simulink model "ECG_test"  (R2020a)
settings: Solver=FixedStepAuto  StartTime=0.0  StopTime=120  FixedStep=1e-3  RelTol=1e-3  EnableMultiTasking=on
undefined symbols (not defined in the file or in its folder): A3, A4, D0, D1, D10, D11, D12, D13, D2, D3, D5, D6, D8, D9, Modes, PTA0, PTA1, PTA2, PTB11, PTB9, PTC11, PTC16, PTC17, PTC2, PTC4, PTD0, PTD1, PTD2, PTD3
libraries: frdmk64flib x15, simulink x1
settings Model: SimulationMode=external  ExtModeTrigDuration=5  Creator=aboda  LastModifiedBy=USER
settings OptimizationCC: EnhancedBackFolding=on  PassReuseOutputArgsAs=Individual arguments  ZeroExternalMemoryAtStartup=off  ZeroInternalMemoryAtStartup=off  MaxStackSize=64  OptimizeBlockOrder=speed  DifferentSizesBufferReuse=on  OptimizationCustomize=off  EfficientTunableParamExpr=on
settings DebuggingCC: ParameterTunabilityLossMsg=error
settings HardwareCC: ProdBitPerPointer=32  ProdBitPerSizeT=32  ProdBitPerPtrDiffT=32  ProdLargestAtomicInteger=Long  ProdLargestAtomicFloat=Double  ProdWordSize=32  ProdHWDeviceType=ARM Compatible->ARM Cortex
settings SFSimCC: MATLABDynamicMemAlloc=off
settings RTWCC: SystemTargetFile=ert.tlc  HardwareBoard=NXP FRDM-K64F  TemplateMakefile=ert_default_tmf  Toolchain=GNU Tools for ARM Embedded Processors
settings CodeAppCC: ForceParamTrailComments=on  IgnoreCustomStorageClasses=off  OperatorAnnotations=on  SimulinkDataObjDesc=on  SFDataObjDesc=on  InsertBlockDesc=on
settings ERTTargetCC: ExtMode=on  ExtModeTransport=4  ExtModeMexFile=sendToCommService  ExtModeMexArgs='ECG_test' 0

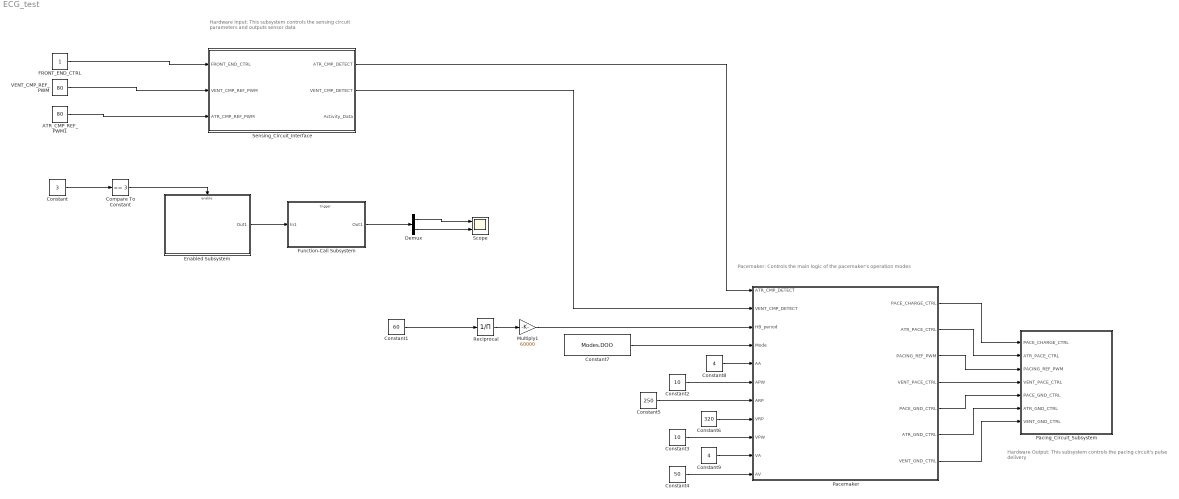
== system ECG_test ==
  note: Hardware Output: This subsystem controls the pacing circuit's pulse delivery
  note: Pacemaker: Controls the main logic of the pacemaker's operation modes
  note: Hardware Input: This subsystem controls the sensing circuit parameters and outputs sensor data
  ATR_CMP_REF_PWM1 : Constant  Value=80  OutDataTypeStr=uint8
  Compare To Constant : simulink/Logic and Bit Operations/Compare To Constant  relop===  const=3  OutDataTypeStr=boolean
  Constant : Constant  Value=3
  Constant1 : Constant  Value=60  OutDataTypeStr=uint8
  Constant2 : Constant  Value=10  OutDataTypeStr=uint8
  Constant3 : Constant  Value=10  OutDataTypeStr=uint8
  Constant4 : Constant  Value=50  OutDataTypeStr=uint16
  Constant5 : Constant  Value=250  OutDataTypeStr=uint16
  Constant6 : Constant  Value=320  OutDataTypeStr=uint16
  Constant7 : Constant  Value=Modes.DOO  OutDataTypeStr=Enum: Modes
  Constant8 : Constant  Value=4  OutDataTypeStr=single
  Constant9 : Constant  Value=4  OutDataTypeStr=single
  Demux : Demux  Outputs=2
  Enabled Subsystem : Subsystem  TreatAsAtomicUnit=on
  FRONT_END_CTRL : Constant  OutDataTypeStr=boolean
  Function-Call Subsystem : Subsystem  TreatAsAtomicUnit=on
  Multiply1 : Gain  Gain=60000  OutDataTypeStr=uint16  RndMeth=Round  SaturateOnIntegerOverflow=on
  Pacemaker : Stateflow chart  TreatAsAtomicUnit=on
      settings: PortSchema="{\"entries\":[{\"content\":{\"sides\":[{\"content\":{\"connectorIds\":[\"In2\",\"In3\",\"In10\",\"In1\",\"In6\",\"In8\",\"In4\",\"In5\",\"In9\",\"In7\",\"In11\"]},\"type\":\"ConnectorPlacement.EquallySpacedRectSide\",\"uuid\":\"be11ab42-f218-4533-b046-48d6c6672980\"},{\"content\":{\"connectorIds\":[\"Out1\",\"Out2\",\"Out3\",\"Out4\",\"Out5\",\"Out6\",\"Out7\"],\"side\":\"RIGHT\"},\"type\":\"ConnectorPlacement.EquallySpacedRectSide\",\"uuid\":\"3184d97a-d95e-4f92-be49-d512e0e8be59\"},{\"content\":{\"connectorIds\":[],\"side\":\"TOP\"},\"type\":\"ConnectorPlacement.EquallySpacedRectSide\",\"uuid\":\"82a667a0-8f6e-4fe8-9d7d-d285af85bcaa\"}]},\"type\":\"ConnectorPlacement.EquallySpacedConnector\",\"uuid\":\"8df3a08e-b350-4a50-854d-64d5d1a667ae\"}],\"packageUris\":[\"http://schema.mathworks.com/mf0/Connector/19700101\"],\"version\":\"1.0\"}"
  Pacing_Circuit_Subsystem : Subsystem
  Reciprocal : Product  Inputs=/  OutDataTypeStr=double  RndMeth=Nearest
  Scope : Scope  NumInputPorts=2
  Sensing_Circuit_Interface : Subsystem
  VENT_CMP_REF_PWM : Constant  Value=80  OutDataTypeStr=uint8
  wires:
  Compare To Constant/1 -> Enabled Subsystem/Enable
  Constant/1 -> Compare To Constant/1
  Enabled Subsystem/1(Out1) -> Function-Call Subsystem/1(In1)
  Function-Call Subsystem/1(Out1) -> Demux/1
  Demux/1 -> Scope/1
  Demux/2 -> Scope/2
  Pacemaker/5(PACE_GND_CTRL) -> Pacing_Circuit_Subsystem/5(PACE_GND_CTRL)
  Pacemaker/1(PACE_CHARGE_CTRL) -> Pacing_Circuit_Subsystem/1(PACE_CHARGE_CTRL)
  Pacemaker/7(VENT_GND_CTRL) -> Pacing_Circuit_Subsystem/7(VENT_GND_CTRL)
  Pacemaker/6(ATR_GND_CTRL) -> Pacing_Circuit_Subsystem/6(ATR_GND_CTRL)
  Pacemaker/4(VENT_PACE_CTRL) -> Pacing_Circuit_Subsystem/4(VENT_PACE_CTRL)
  Pacemaker/2(ATR_PACE_CTRL) -> Pacing_Circuit_Subsystem/2(ATR_PACE_CTRL)
  Pacemaker/3(PACING_REF_PWM) -> Pacing_Circuit_Subsystem/3(PACING_REF_PWM)
  ATR_CMP_REF_PWM1/1 -> Sensing_Circuit_Interface/3(ATR_CMP_REF_PWM)
  VENT_CMP_REF_PWM/1 -> Sensing_Circuit_Interface/2(VENT_CMP_REF_PWM)
  FRONT_END_CTRL/1 -> Sensing_Circuit_Interface/1(FRONT_END_CTRL)
  Sensing_Circuit_Interface/1(ATR_CMP_DETECT) -> Pacemaker/2(ATR_CMP_DETECT)
  Sensing_Circuit_Interface/2(VENT_CMP_DETECT) -> Pacemaker/3(VENT_CMP_DETECT)
  Constant3/1 -> Pacemaker/9(VPW)
  Constant4/1 -> Pacemaker/11(AV)
  Constant5/1 -> Pacemaker/4(ARP)
  Constant6/1 -> Pacemaker/5(VRP)
  Constant2/1 -> Pacemaker/8(APW)
  Constant7/1 -> Pacemaker/1(Mode)
  Constant8/1 -> Pacemaker/6(AA)
  Constant9/1 -> Pacemaker/7(VA)
  Reciprocal/1 -> Multiply1/1
  Constant1/1 -> Reciprocal/1
  Multiply1/1 -> Pacemaker/10(HB_period)

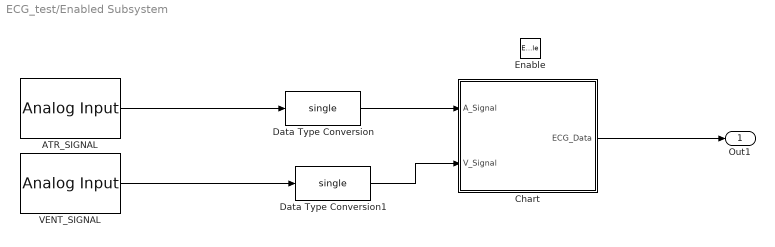
== system ECG_test/Enabled Subsystem ==
  Enable : EnablePort
  ATR_SIGNAL : frdmk64flib/Analog Input  Whichpin=PTB11 (A3)  SampleTime=-1
  Chart : Stateflow chart  TreatAsAtomicUnit=on
  Data Type Conversion : DataTypeConversion  OutDataTypeStr=single
  Data Type Conversion1 : DataTypeConversion  OutDataTypeStr=single
  VENT_SIGNAL : frdmk64flib/Analog Input  Whichpin=PTC11 (A4)  SampleTime=-1
  Out1 : Outport
  wires:
  Chart/1(ECG_Data) -> Out1/1
  Data Type Conversion/1 -> Chart/1(A_Signal)
  Data Type Conversion1/1 -> Chart/2(V_Signal)
  ATR_SIGNAL/1 -> Data Type Conversion/1
  VENT_SIGNAL/1 -> Data Type Conversion1/1

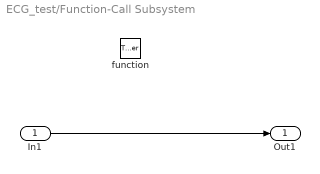
== system ECG_test/Function-Call Subsystem ==
  In1 : Inport
  function : TriggerPort  TriggerType=function-call  IsSimulinkFunction=on  FunctionName=Send_Params  VariantControl=Variant
  Out1 : Outport
  wires:
  In1/1 -> Out1/1

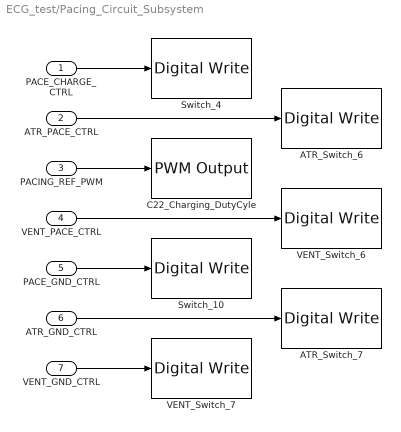
== system ECG_test/Pacing_Circuit_Subsystem ==
  PACE_CHARGE_CTRL : Inport  OutDataTypeStr=boolean
  ATR_PACE_CTRL : Inport  Port=2  OutDataTypeStr=boolean
  PACING_REF_PWM : Inport  Port=3  OutDataTypeStr=uint8
  VENT_PACE_CTRL : Inport  Port=4  OutDataTypeStr=boolean
  PACE_GND_CTRL : Inport  Port=5  OutDataTypeStr=boolean
  ATR_GND_CTRL : Inport  Port=6  OutDataTypeStr=boolean
  VENT_GND_CTRL : Inport  Port=7  OutDataTypeStr=boolean
  ATR_Switch_6 : frdmk64flib/Digital Write  Whichpin=PTA0 (D8)
  ATR_Switch_7 : frdmk64flib/Digital Write  Whichpin=PTD2 (D11)
  C22_Charging_DutyCyle : frdmk64flib/PWM Output  Whichpin=PTA2 (D5)  InitialFrequency=2000  InitialDutyCycle=0
  Switch_10 : frdmk64flib/Digital Write  Whichpin=PTD0 (D10)
  Switch_4 : frdmk64flib/Digital Write  Whichpin=PTB9 (D2)
  VENT_Switch_6 : frdmk64flib/Digital Write  Whichpin=PTC4 (D9)
  VENT_Switch_7 : frdmk64flib/Digital Write  Whichpin=PTD3 (D12)
  wires:
  ATR_PACE_CTRL/1 -> ATR_Switch_6/1
  PACING_REF_PWM/1 -> C22_Charging_DutyCyle/1
  VENT_PACE_CTRL/1 -> VENT_Switch_6/1
  PACE_CHARGE_CTRL/1 -> Switch_4/1
  PACE_GND_CTRL/1 -> Switch_10/1
  VENT_GND_CTRL/1 -> VENT_Switch_7/1
  ATR_GND_CTRL/1 -> ATR_Switch_7/1

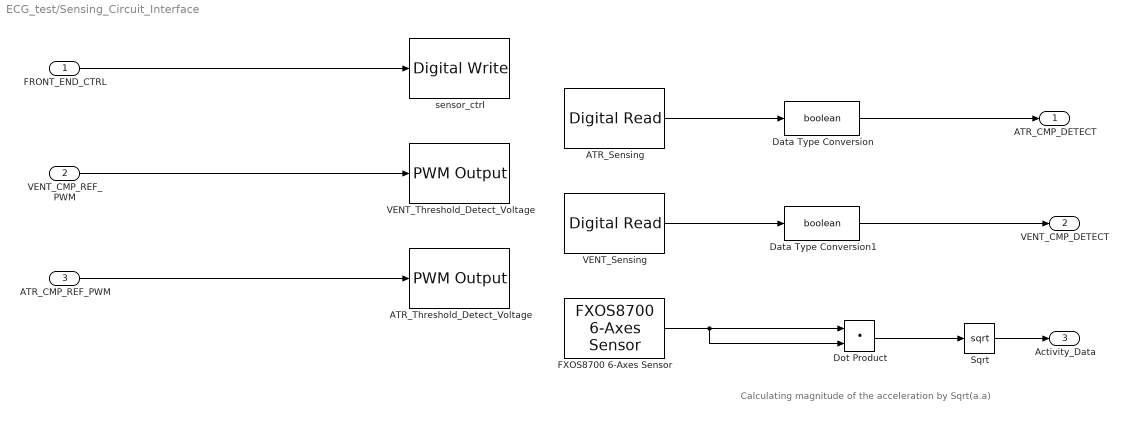
== system ECG_test/Sensing_Circuit_Interface ==
  note: Calculating magnitude of the acceleration by Sqrt(a.a)
  FRONT_END_CTRL : Inport  OutDataTypeStr=boolean
  VENT_CMP_REF_PWM : Inport  Port=2  OutDataTypeStr=uint8
  ATR_CMP_REF_PWM : Inport  Port=3  OutDataTypeStr=uint8
  ATR_Sensing : frdmk64flib/Digital Read  Whichpin=PTC16 (D0)  SampleTime=-1
  ATR_Threshold_Detect_Voltage : frdmk64flib/PWM Output  Whichpin=PTC2 (D6)  InitialFrequency=2000  InitialDutyCycle=0
  Data Type Conversion : DataTypeConversion  OutDataTypeStr=boolean
  Data Type Conversion1 : DataTypeConversion  OutDataTypeStr=boolean
  Dot Product : DotProduct  OutDataTypeStr=double  InputSameDT=on
  FXOS8700 6-Axes Sensor : frdmk64flib/FXOS8700 6-Axes Sensor  Activesensor=Accelerometer only  ODR=800Hz  HybridODR=400Hz  Accelfullrange=-4g to +4g  SampleTime=-1
  Sqrt : Sqrt  OutDataTypeStr=double  SaturateOnIntegerOverflow=on
  VENT_Sensing : frdmk64flib/Digital Read  Whichpin=PTC17 (D1)  SampleTime=-1
  VENT_Threshold_Detect_Voltage : frdmk64flib/PWM Output  Whichpin=PTA1 (D3)  InitialFrequency=2000  InitialDutyCycle=0
  sensor_ctrl : frdmk64flib/Digital Write  Whichpin=PTD1 (D13)
  ATR_CMP_DETECT : Outport  OutDataTypeStr=boolean
  VENT_CMP_DETECT : Outport  Port=2  OutDataTypeStr=boolean
  Activity_Data : Outport  Port=3  OutDataTypeStr=double
  wires:
  VENT_Sensing/1 -> Data Type Conversion1/1
  ATR_Sensing/1 -> Data Type Conversion/1
  ATR_CMP_REF_PWM/1 -> ATR_Threshold_Detect_Voltage/1
  FRONT_END_CTRL/1 -> sensor_ctrl/1
  VENT_CMP_REF_PWM/1 -> VENT_Threshold_Detect_Voltage/1
  Data Type Conversion/1 -> ATR_CMP_DETECT/1
  Data Type Conversion1/1 -> VENT_CMP_DETECT/1
  Dot Product/1 -> Sqrt/1
  FXOS8700 6-Axes Sensor/1 -> Dot Product/2, Dot Product/1
  Sqrt/1 -> Activity_Data/1

== stateflow chart ECG_test/Pacemaker ==
  state AOO
    state Initial_ATR
      entry:
      % Charging C22 and Discharging C21
      ATR_PACE_CTRL = false;
      VENT_PACE_CTRL = false;
      PACING_REF_PWM = cast(AA*100/5,'uint8');
      PACE_CHARGE_CTRL = true;
      PACE_GND_CTRL = true;
      VENT_GND_CTRL = false;
      ATR_GND_CTRL = true;
      inPace = false;
    state Pace_ATR
      %This subchart is responsible for pacing the atrium
      state ATR_Pacing
        entry:
        %Discharging C22 through the heart
        PACE_CHARGE_CTRL = false;
        ATR_GND_CTRL = false;
        ATR_PACE_CTRL = true;
        inPace = true;
      state Charge_PaceC_Discharge_BlockingC
        entry:
        %Charging C22 and Discharging C21
        %Setting PACING_REF PWM is not needed since
        %it didn't change from the initial state
        ATR_PACE_CTRL = false;
        VENT_PACE_CTRL = false;
        PACE_CHARGE_CTRL = true;
        PACE_GND_CTRL = true;
        VENT_GND_CTRL = false;
        ATR_GND_CTRL = true;
        inPace = false;
      (default) -> AOO.Pace_ATR.ATR_Pacing
      AOO.Pace_ATR.ATR_Pacing -> AOO.Pace_ATR.Charge_PaceC_Discharge_BlockingC : after(APW,msec)
    note: Initial delay to charge C22
    (default) -> AOO.Initial_ATR
    AOO.Initial_ATR -> AOO.Pace_ATR : after(HB_period,msec)
    AOO.Pace_ATR -> AOO.Pace_ATR : after(HB_period,msec)
  note: Pace_ATR and Pace_VENT are subcharts which are responsible for delivering a single artificial pulse to the atrium and ventricle respectively
  state VOO
    state Initial_VENT
      entry:
      %Charging C22 and Discharging C21
      ATR_PACE_CTRL = false;
      VENT_PACE_CTRL = false;
      PACING_REF_PWM = cast(VA*100/5,'uint8');
      PACE_CHARGE_CTRL = true;
      PACE_GND_CTRL = true;
      ATR_GND_CTRL = false;
      VENT_GND_CTRL = true;
      inPace = false;
    note: Initial delay to charge C22
    state Pace_VENT
      %This subchart is for pacing the ventricle
      state VENT_Pacing
        entry:
        %Discharging C22 through the heart
        PACE_CHARGE_CTRL=false;
        VENT_GND_CTRL=false;
        VENT_PACE_CTRL=true;
        inPace = true;
      state Charge_PaceC_Discharge_Discharge_BlockingC
        entry:
        %Charging C22 and Discharging C21
        %Setting PACING_REF PWM is not needed since
        %it didn't change from the initial state
        ATR_PACE_CTRL = false;
        VENT_PACE_CTRL = false;
        PACE_CHARGE_CTRL = true;
        PACE_GND_CTRL = true;
        ATR_GND_CTRL=false;
        VENT_GND_CTRL = true;
        inPace = false;
      (default) -> VOO.Pace_VENT.VENT_Pacing
      VOO.Pace_VENT.VENT_Pacing -> VOO.Pace_VENT.Charge_PaceC_Discharge_Discharge_BlockingC : after(VPW,msec)
    (default) -> VOO.Initial_VENT
    VOO.Initial_VENT -> VOO.Pace_VENT : after(HB_period,msec)
    VOO.Pace_VENT -> VOO.Pace_VENT : after(HB_period,msec)
  state No_Pace
    %Setting default values of parameters
    PACE_CHARGE_CTRL = false;
    ATR_PACE_CTRL = false;
    PACING_REF_PWM = 0;
    VENT_PACE_CTRL = false;
    PACE_GND_CTRL = true;
    ATR_GND_CTRL = true;
    VENT_GND_CTRL = true;
    inPace = false;
    %HB_period = 1000/(cast(LRL,'uint16')/60);
  note: The inPace variable is used to avoid switching modes while delivering a pace (explained in pacemaker documentation)
  state VVI
    state Initial_VENT
      entry:
      %Charging C22 and Discharging C21
      ATR_PACE_CTRL = false;
      VENT_PACE_CTRL = false;
      PACING_REF_PWM = cast(VA*100/5,'uint8');
      PACE_CHARGE_CTRL = true;
      PACE_GND_CTRL = true;
      ATR_GND_CTRL = false;
      VENT_GND_CTRL = true;
      inPace = false;
    state Sense
      %{
      In this state we wait to sense a natural pulse from
      the heart. If the heart sends a pulse within
      (heart beat period - refractory period), we
      send inhibit the pace and go to the wait state.
      Else, we send an artificial pulse to the heart
      %}
    state wait_NP
      %{
      We enter this state if we
      detect a natural pulse from
      the heart and ignore all
      incoming heart signals for the
      duration of the refractory period
      %}
    state Pace_VENT
      %This subchart is for pacing the ventricle
      state VENT_Pacing
        entry:
        %Discharging C22 through the heart
        PACE_CHARGE_CTRL=false;
        VENT_GND_CTRL=false;
        VENT_PACE_CTRL=true;
        inPace = true;
      state Charge_PaceC_Discharge_Discharge_BlockingC
        entry:
        %Charging C22 and Discharging C21
        %Setting PACING_REF PWM is not needed since
        %it didn't change from the initial state
        ATR_PACE_CTRL = false;
        VENT_PACE_CTRL = false;
        PACE_CHARGE_CTRL = true;
        PACE_GND_CTRL = true;
        ATR_GND_CTRL=false;
        VENT_GND_CTRL = true;
        inPace = false;
      (default) -> VVI.Pace_VENT.VENT_Pacing
      VVI.Pace_VENT.VENT_Pacing -> VVI.Pace_VENT.Charge_PaceC_Discharge_Discharge_BlockingC : after(VPW,msec)
    VVI.Sense -> VVI.wait_NP [order 1] : [VENT_CMP_DETECT == true]
    (default) -> VVI.Initial_VENT
    VVI.wait_NP -> VVI.Sense : after(VRP,msec)
    VVI.Initial_VENT -> VVI.Sense
    VVI.Sense -> VVI.Pace_VENT [order 2] : after(HB_period-VRP,msec)
    VVI.Pace_VENT -> VVI.Sense : after(VRP,msec)
  state AAI
    state Initial_ATR
      entry:
      % Charging C22 and Discharging C21
      ATR_PACE_CTRL = false;
      VENT_PACE_CTRL = false;
      PACING_REF_PWM = cast(AA*100/5,'uint8');
      PACE_CHARGE_CTRL = true;
      PACE_GND_CTRL = true;
      VENT_GND_CTRL = false;
      ATR_GND_CTRL = true;
      inPace = false;
    state Sense
      %{
      In this state we wait to sense a natural pulse from
      the heart. If the heart sends a pulse within
      (heart beat period - refractory period), we
      send inhibit the pace and go to the wait state.
      Else, we send an artificial pulse to the heart
      %}
    state wait_NP
      %{
      We enter this state if we
      detect a natural pulse from
      the heart and ignore all
      incoming heart signals for the
      duration of the refractory period
      %}
    state Pace_ATR
      %This subchart is responsible for pacing the atrium
      state ATR_Pacing
        entry:
        %Discharging C22 through the heart
        PACE_CHARGE_CTRL = false;
        ATR_GND_CTRL = false;
        ATR_PACE_CTRL = true;
        inPace = true;
      state Charge_PaceC_Discharge_BlockingC
        entry:
        %Charging C22 and Discharging C21
        %Setting PACING_REF PWM is not needed since
        %it didn't change from the initial state
        ATR_PACE_CTRL = false;
        VENT_PACE_CTRL = false;
        PACE_CHARGE_CTRL = true;
        PACE_GND_CTRL = true;
        VENT_GND_CTRL = false;
        ATR_GND_CTRL = true;
        inPace = false;
      (default) -> AAI.Pace_ATR.ATR_Pacing
      AAI.Pace_ATR.ATR_Pacing -> AAI.Pace_ATR.Charge_PaceC_Discharge_BlockingC : after(APW,msec)
    (default) -> AAI.Initial_ATR
    AAI.Sense -> AAI.wait_NP [order 2] : [ATR_CMP_DETECT == true]
    AAI.Initial_ATR -> AAI.Sense
    AAI.wait_NP -> AAI.Sense : after(ARP,msec)
    AAI.Sense -> AAI.Pace_ATR [order 1] : after(HB_period - ARP,msec)
    AAI.Pace_ATR -> AAI.Sense : after(ARP,msec)
  state DOO
    state Initial_ATR
      entry:
      % Charging C22 and Discharging C21
      ATR_PACE_CTRL = false;
      VENT_PACE_CTRL = false;
      PACING_REF_PWM = cast(AA*100/5,'uint8');
      PACE_CHARGE_CTRL = true;
      PACE_GND_CTRL = true;
      VENT_GND_CTRL = false;
      ATR_GND_CTRL = true;
      inPace = false;
    state Pace_ATR
      %This subchart is responsible for pacing the atrium
      state ATR_Pacing
        entry:
        %Discharging C22 through the heart
        PACE_CHARGE_CTRL = false;
        ATR_GND_CTRL = false;
        ATR_PACE_CTRL = true;
        inPace = true;
      state Initial_VENT
        entry:
        %Charging C22 and Discharging C21
        ATR_PACE_CTRL = false;
        VENT_PACE_CTRL = false;
        PACING_REF_PWM = cast(VA*100/5,'uint8');
        PACE_CHARGE_CTRL = true;
        PACE_GND_CTRL = true;
        ATR_GND_CTRL = false;
        VENT_GND_CTRL = true;
        inPace = false;
      (default) -> DOO.Pace_ATR.ATR_Pacing
      DOO.Pace_ATR.ATR_Pacing -> DOO.Pace_ATR.Initial_VENT : after(APW,msec)
    state Pace_VENT
      %This subchart is for pacing the ventricle
      state VENT_Pacing
        entry:
        %Discharging C22 through the heart
        PACE_CHARGE_CTRL=false;
        VENT_GND_CTRL=false;
        VENT_PACE_CTRL=true;
        inPace = true;
      state Charge_PaceC_Discharge_BlockingC
        entry:
        %Charging C22 and Discharging C21
        %Setting PACING_REF PWM is not needed since
        %it didn't change from the initial state
        ATR_PACE_CTRL = false;
        VENT_PACE_CTRL = false;
        PACE_CHARGE_CTRL = true;
        PACE_GND_CTRL = true;
        VENT_GND_CTRL = false;
        ATR_GND_CTRL = true;
        inPace = false;
      (default) -> DOO.Pace_VENT.VENT_Pacing
      DOO.Pace_VENT.VENT_Pacing -> DOO.Pace_VENT.Charge_PaceC_Discharge_BlockingC : after(VPW,msec)
    (default) -> DOO.Initial_ATR
    DOO.Initial_ATR -> DOO.Pace_ATR : after(HB_period-AV,msec)
    DOO.Pace_VENT -> DOO.Pace_ATR : after(HB_period-AV,msec)
    DOO.Pace_ATR -> DOO.Pace_VENT : after(AV,msec)
  (default) -> No_Pace
  (junction 22) -> AOO [order 3] : [Mode == Modes.AOO]
  AOO -> (junction 22) : [Mode ~=Modes.AOO && inPace == false]
  VOO -> (junction 22) : [Mode ~= Modes.VOO  && inPace == false]
  No_Pace -> (junction 22) : [Mode ~= Modes.NO_PACE]
  (junction 22) -> VOO [order 4] : [Mode == Modes.VOO]
  (junction 22) -> No_Pace [order 1] : [Mode == Modes.NO_PACE]
  (junction 22) -> VVI [order 5] : [Mode == Modes.VVI]
  (junction 22) -> AAI [order 6] : [Mode == Modes.AAI]
  AAI -> (junction 22) : [Mode ~= Modes.AAI  && inPace == false]
  (junction 22) -> DOO [order 2] : [Mode==Modes.DOO]
  DOO -> (junction 22) : [Mode ~= Modes.DOO && inPace == false]
  VVI -> (junction 22) : [Mode ~= Modes.VVI  && inPace == false]
  data: Mode input Enum: Modes; ATR_CMP_DETECT input boolean; VENT_CMP_DETECT input boolean; ARP input uint16; VRP input uint16; AA input single; VA input single; APW input uint8; VPW input uint8; PACE_CHARGE_CTRL output boolean; ATR_PACE_CTRL output boolean; PACING_REF_PWM output uint8; VENT_PACE_CTRL output boolean; PACE_GND_CTRL output boolean; ATR_GND_CTRL output boolean; VENT_GND_CTRL output boolean; HB_period input uint16; AV input uint16; inPace local boolean

== stateflow chart ECG_test/Enabled Subsystem/Chart ==
  state Sampling
    en:
    ECG_Data(counter) = A_Signal;
    ECG_Data(counter+20) = V_Signal;
    counter = counter + 1;
  state Initialize
    en:
    ECG_Data = zeros(1,40);
    counter = 1;
    sampling_interval = 2;
  (default) -> Initialize
  Sampling -> Sampling [order 2] : after(sampling_interval,msec)
  Initialize -> Sampling
  Sampling -> Initialize [order 1] : [counter == 21]{Send_Params();}
  data: A_Signal input single; V_Signal input single; ECG_Data output single size=[1,40]; sampling_interval local uint16; counter local uint8
